simulink model "AI_HW01_Q03"  (R2022a)
settings: Solver=VariableStepAuto  StartTime=0.0  StopTime=10.0  RelTol=1e-3
undefined symbols (not defined in the file or in its folder): A, B, C, D
libraries: fuzblock x1
settings Model: Creator=Arash  LastModifiedBy=Arash

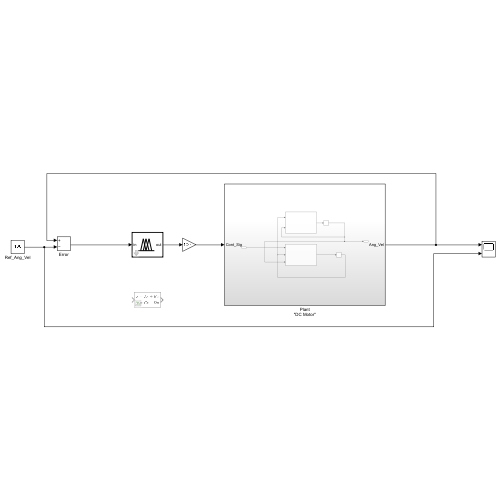
[thumbnail: Simulink's stored preview of the top-level diagram]
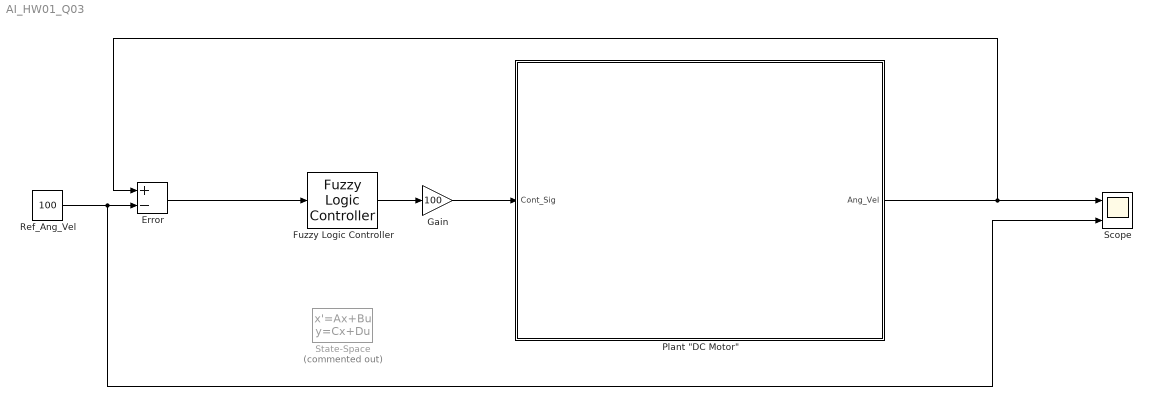
== system AI_HW01_Q03 ==
  Error : Sum  Inputs=+-
  Fuzzy Logic Controller : fuzblock/Fuzzy Logic  Controller  FIS='Newone.fis'  OutputSampleNumber=101  DataType=double  FuzzifiedInputs=off  RuleFiringStrengths=off  RuleOutputs=off  AggregatedOutputs=off  SimulateUsing=Interpreted execution  OutOfRangeInputValueMessage=warning  NoRuleFiredMessage=warning  EmptyOutputFuzzySetMessage=warning
  Gain : Gain  Gain=100
  "Plant \"DC Motor\"" : Subsystem
  Ref_Ang_Vel : Constant  Value=100
  Scope : Scope  NumInputPorts=2
  State-Space : StateSpace  Commented=on  A=A  B=B  C=C  D=D  InitialCondition=0
  wires:
  Fuzzy Logic Controller/1 -> Gain/1
  Ref_Ang_Vel/1 -> Scope/2, Error/2
  Error/1 -> Fuzzy Logic Controller/1
  Gain/1 -> "Plant \"DC Motor\""/1(Cont_Sig)
  "Plant \"DC Motor\""/1(Ang_Vel) -> Error/1, Scope/1

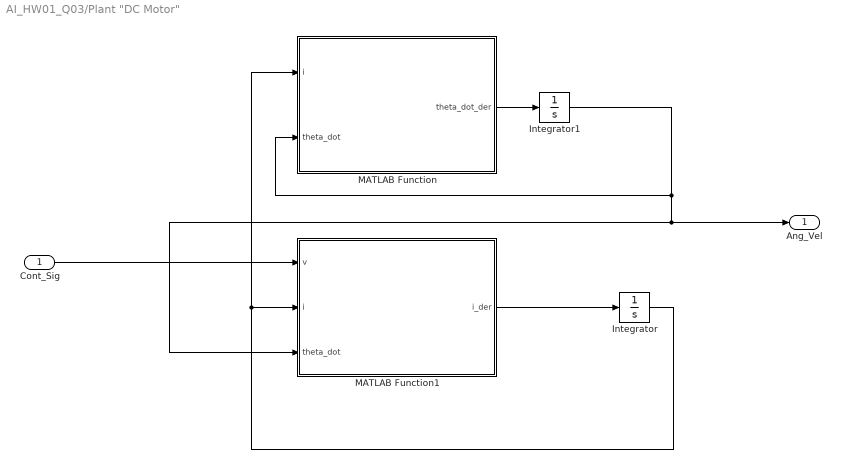
== system AI_HW01_Q03/Plant "DC Motor" ==
  Cont_Sig : Inport
  Integrator : Integrator
  Integrator1 : Integrator
  MATLAB Function : MATLAB Function  TreatAsAtomicUnit=on
  MATLAB Function1 : MATLAB Function  TreatAsAtomicUnit=on
  Ang_Vel : Outport
  wires:
  MATLAB Function/1(theta_dot_der) -> Integrator1/1
  MATLAB Function1/1(i_der) -> Integrator/1
  Integrator1/1 -> MATLAB Function/2(theta_dot), MATLAB Function1/3(theta_dot), Ang_Vel/1
  Integrator/1 -> MATLAB Function/1(i), MATLAB Function1/2(i)
  Cont_Sig/1 -> MATLAB Function1/1(v)

== matlab function AI_HW01_Q03/Plant "DC Motor"/MATLAB Function ==
  data: i input; theta_dot input; theta_dot_der output
function theta_dot_der = DCMotor(i, theta_dot)

K = 0.01;
J = 0.01;
b = 0.1;
L = 0.5;
R = 1;

theta_dot_der = (-b/J) * theta_dot + (K/J) * i;      % theta_double_dot

end

== matlab function AI_HW01_Q03/Plant "DC Motor"/MATLAB Function1 ==
  data: v input; i input; theta_dot input; i_der output
function i_der = DCMotor(v, i, theta_dot)

K = 0.01;
J = 0.01;
b = 0.1;
L = 0.5;
R = 1;

i_der = (-K/J) * theta_dot - (R/L) * i + (1/L) * v;     % i_dot

end
